simulink model "Bai29"  (R2020a)
settings: Solver=VariableStepAuto  StartTime=0.1  StopTime=10  RelTol=1e-3
settings Model: Creator=NgocNguyen  LastModifiedBy=NgocNguyen

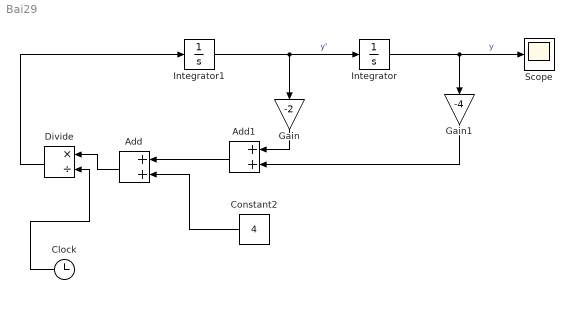
== system Bai29 ==
  Add : Sum
  Add1 : Sum
  Clock : Clock
      settings: Decimation=100
  Constant2 : Constant  Value=4
  Divide : Product  Inputs=*/
  Gain : Gain  Gain=-2
  Gain1 : Gain  Gain=-4
  Integrator : Integrator  InitialCondition=1
  Integrator1 : Integrator  InitialCondition=1
  Scope : Scope
  wires:
  Integrator1/1 -> Gain/1, Integrator/1  "y'"
  Integrator/1 -> Scope/1, Gain1/1  "y"
  Gain/1 -> Add1/1
  Gain1/1 -> Add1/2
  Add1/1 -> Add/1
  Constant2/1 -> Add/2
  Divide/1 -> Integrator1/1
  Add/1 -> Divide/1
  Clock/1 -> Divide/2
